simulink model "pendulo"  (R2025b)
settings: Solver=VariableStepAuto  StartTime=0.0  StopTime=10.0  RelTol=1e-3
settings Model: Creator=leona  LastModifiedBy=leona

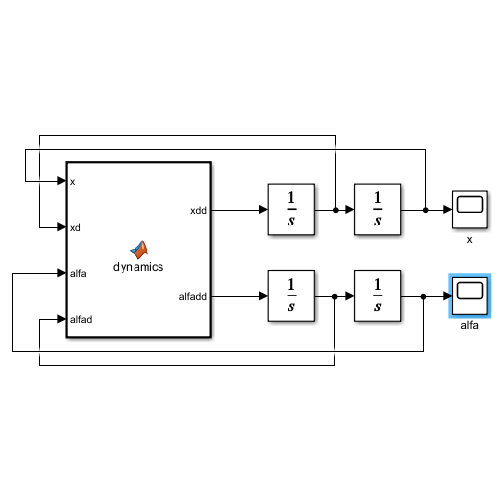
[thumbnail: Simulink's stored preview of the top-level diagram]
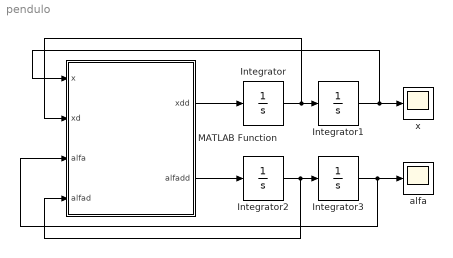
== system pendulo ==
  Integrator : Integrator
  Integrator1 : Integrator
  Integrator2 : Integrator
  Integrator3 : Integrator  InitialCondition=0.01745329252
  MATLAB Function : MATLAB Function  TreatAsAtomicUnit=on
  alfa : Scope
      settings: ActiveDisplayYMinimum=-0.63347576854003085  ActiveDisplayYMaximum=5.8758148420602785
  x : Scope
      settings: ActiveDisplayYMinimum=-0.098370042474869884  ActiveDisplayYMaximum=0.096333497674656585
  wires:
  MATLAB Function/1(xdd) -> Integrator/1
  MATLAB Function/2(alfadd) -> Integrator2/1
  Integrator2/1 -> MATLAB Function/4(alfad), Integrator3/1
  Integrator1/1 -> MATLAB Function/1(x), x/1
  Integrator3/1 -> MATLAB Function/3(alfa), alfa/1
  Integrator/1 -> MATLAB Function/2(xd), Integrator1/1

== matlab function pendulo/MATLAB Function ==
  data: x input; xdd output; xd input; alfa input; alfad input; alfadd output
function [xdd, alfadd] = dynamics(x, xd, alfa, alfad)

ip = 0.0079;
mc = 0.7031;
lp = 0.3302;
mp = 0.23;
fc = 0;
beq = 4.3;
g  = 9.81;
bp = 0.0024;
xdd = 0;
alfadd = 0;

denominador = (mc+mp)*ip + mc*mp*lp^2 + mp^2*lp^2*sin(alfa)^2;

xdd = ( (ip + mp*lp^2)*fc + mp^2*lp^2*g*cos(alfa)*sin(alfa) - (ip + mp*lp^2)*beq*xd - mp*lp*(ip + mp*lp^2)*alfad^2*sin(alfa) - mp*lp*bp*alfad*cos(alfa) ) / denominador;

alfadd = ( (mc + mp)*mp*g*lp*sin(alfa) - (mc + mp)*bp*alfad + fc*mp*lp*cos(alfa) - mp^2*lp^2*alfad^2*sin(alfa)*cos(alfa) - beq*mp*lp*xd*cos(alfa) ) / denominador;

end
